simulink model "TransmissionController"  (R2022b)
settings: configuration reference "VehicleFixed10ms" (kept outside this file)
StartFcn:
  | %tic
StopFcn:
  | %toc
libraries: autolibtranscontrolscommon x1
settings Model: DataDictionary=VirtualVehicleTemplate.sldd  ModifiedByFormat=The MathWorks, Inc.  Creator=The MathWorks, Inc.  LastModifiedBy=The MathWorks, Inc.
settings ConfigSetRef: SourceName=VehicleFixed10ms

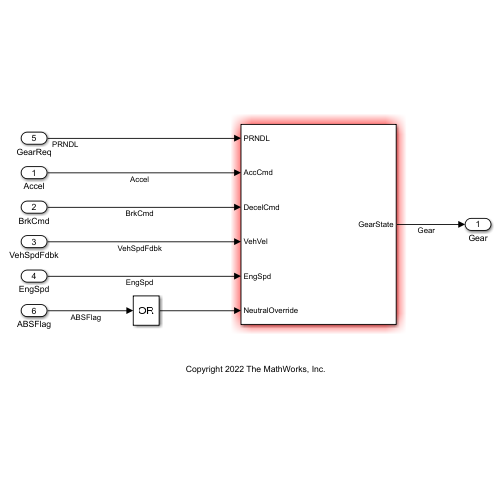
[thumbnail: Simulink's stored preview of the top-level diagram]
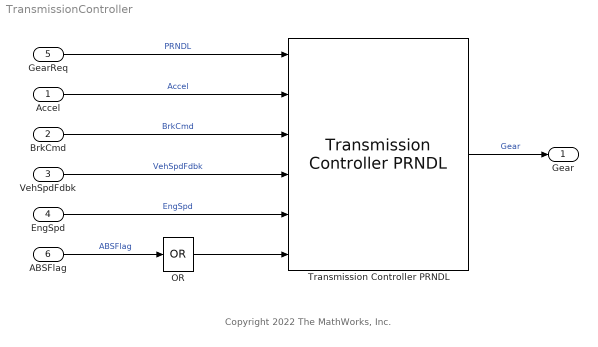
== system TransmissionController ==
  note: Copyright 2022 The MathWorks, Inc.
  Accel : Inport  OutDataTypeStr=double  PortDimensions=1
  BrkCmd : Inport  Port=2  OutDataTypeStr=double  PortDimensions=1
  VehSpdFdbk : Inport  Port=3  OutDataTypeStr=double  Unit=m/s  PortDimensions=1
  EngSpd : Inport  Port=4  OutDataTypeStr=double  Unit=rad/s  PortDimensions=1
  GearReq : Inport  Port=5  OutDataTypeStr=double  PortDimensions=1
  ABSFlag : Inport  Port=6  OutDataTypeStr=boolean  PortDimensions=4
  OR : Logic  Operator=OR  Inputs=1  AllPortsSameDT=off  OutDataTypeStr=boolean
  Transmission Controller PRNDL : autolibtranscontrolscommon/Transmission Controller PRNDL  ShPattern=Economy  GearInit=CtrlTcuInitGear  LugSpd=CtrlTcuLugSpd  MinUpSpd=CtrlTcuMinUpSpd  tClutchUp=CtrlTcuTmUpSh  tClutchDn=CtrlTcuTmDnSh  tPark=120  VelUnit=km/hr  UpShSpd=CtrlTcuUpShSpd  UpLdBpt=CtrlTcuUpLdBpt  UpShBpt=1:7  DnShSpd=CtrlTcuDnShSpd  DnLdBpt=CtrlTcuDnLdBpt  DnShBpt=2:8  POFS=zeros(4,1)  GOFS=zeros(1,7)  Ngears=8  aMode=6  MaxPwrMode=off  UpShSpd_MaxPwr="[35.619930749150555\t48.3185789489240349\t57.5983603256815684\t70.2526076576236846\t88.5309649148733797\t138.79644737231007\t214.194671058465104;40.119930749150555\t52.8185789489240349\t62.0983603256815684\t74.7526076576236846\t93.0309649148733797\t143.29644737231007\t218.694671058465104;41.619930749150555\t54.3185789489240349\t63.5983603256815684\t76.2526076576236846\t94.5309649148733797\t144.79644737231007\t220.194671058465104;47.619930749150555\t60.3185789489240349\t69.5983603256815684\t82.2526076576236846\t100.53096491487338\t150.79644737231007\t226.194671058465104]"  UpLdBpt_MaxPwr=[0.1 0.4 0.5 0.9]  UpShBpt_MaxPwr=1:7  DnShSpd_MaxPwr="[31.619930749150555\t44.3185789489240349\t53.5983603256815684\t66.2526076576236846\t84.5309649148733797\t134.79644737231007\t210.194671058465104;36.119930749150555\t48.8185789489240349\t58.0983603256815684\t70.7526076576236846\t89.0309649148733797\t139.29644737231007\t214.694671058465104;37.619930749150555\t50.3185789489240349\t59.5983603256815684\t72.2526076576236846\t90.5309649148733797\t140.79644737231007\t216.194671058465104;43.619930749150555\t56.3185789489240349\t65.5983603256815684\t78.2526076576236846\t96.5309649148733797\t146.79644737231007\t222.194671058465104]"  DnLdBpt_MaxPwr=[0.1 0.4 0.5 0.9]  DnShBpt_MaxPwr=2:8  POFS_MaxPwr=zeros(4,1)  GOFS_MaxPwr=zeros(1,7)
  Gear : Outport  OutDataTypeStr=double  PortDimensions=1  VectorParamsAs1DForOutWhenUnconnected=off
  wires:
  ABSFlag/1 -> OR/1  "ABSFlag"
  Transmission Controller PRNDL/1 -> Gear/1  "Gear"
  GearReq/1 -> Transmission Controller PRNDL/1  "PRNDL"
  Accel/1 -> Transmission Controller PRNDL/2  "Accel"
  BrkCmd/1 -> Transmission Controller PRNDL/3  "BrkCmd"
  EngSpd/1 -> Transmission Controller PRNDL/5  "EngSpd"
  VehSpdFdbk/1 -> Transmission Controller PRNDL/4  "VehSpdFdbk"
  OR/1 -> Transmission Controller PRNDL/6
